simulink model "Model2_inout"  (R2023a)
settings: Solver=VariableStepAuto  StartTime=0.0  StopTime=10.0  RelTol=1e-3
undefined symbols (not defined in the file or in its folder): param
settings Model: Creator=Admin  LastModifiedBy=Admin

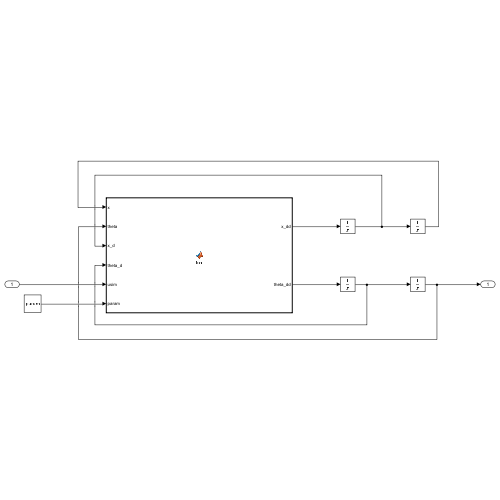
[thumbnail: Simulink's stored preview of the top-level diagram]
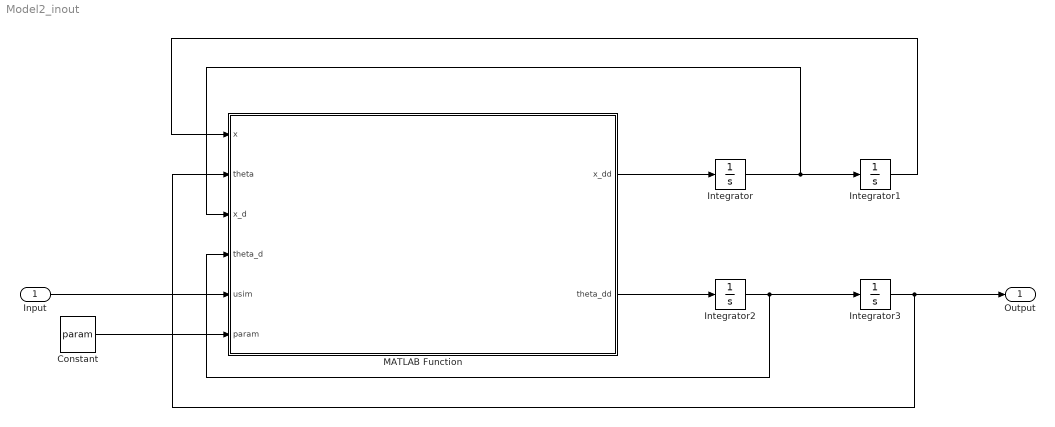
== system Model2_inout ==
  Input : Inport
  Constant : Constant  Value=param  OutDataTypeStr=Bus: par_bus
  Integrator{,1..3} (4 alike) : Integrator
  MATLAB Function : MATLAB Function  TreatAsAtomicUnit=on
  Output : Outport
  wires:
  Constant/1 -> MATLAB Function/6(param)
  MATLAB Function/1(x_dd) -> Integrator/1
  MATLAB Function/2(theta_dd) -> Integrator2/1
  Integrator/1 -> MATLAB Function/3(x_d), Integrator1/1
  Integrator1/1 -> MATLAB Function/1(x)
  Integrator2/1 -> Integrator3/1, MATLAB Function/4(theta_d)
  Integrator3/1 -> MATLAB Function/2(theta), Output/1
  Input/1 -> MATLAB Function/5(usim)

== matlab function Model2_inout/MATLAB Function ==
  data: x input; x_dd output; theta input; x_d input; theta_d input; usim input; param input; theta_dd output
function [x_dd, theta_dd] = fcn(x, theta, x_d, theta_d, usim, param)
x_dd = (param.l0 + x)*theta_d^2 - (param.k/param.m)*x + param.g*cos(theta) - param.csi*x_d;
theta_dd = (-param.g/(param.l0 + x))*sin(theta) - ((2*x_d)/(param.l0 + x))*theta_d - param.csi*theta_d + usim/(param.m*((param.l0+x)^2)); 
end
